simulink model "car_sim_for_student_r2015"  (R2022b)
settings: Solver=FixedStepAuto  StartTime=0.0  StopTime=40  FixedStep=0.001  RelTol=1e-3
InitFcn:
  | load('traj\traj_diySYSU.mat');
  | load('traj\sysu_standard.mat');
  | run lqr_nums.m
StopFcn:
  | run stopFunc.m
values from neighbouring files (symbols this model uses):
  k = lqr(A,B,Q,R)    [lqr_nums.m]
  map = ~map    [stopFunc.m]
undefined symbols (not defined in the file or in its folder): gray, out, trajSYSU
libraries: simulink x3, slpidlib x1
settings Model: Creator=Manny  LastModifiedBy=秦华谦
settings SolverCC: AlgebraicLoopSolver=LineSearch
settings OptimizationCC: LifeSpan=inf
settings DebuggingCC: UnconnectedInputMsg=warning  UnconnectedOutputMsg=warning  UnconnectedLineMsg=warning  SFExecutionAtInitializationDiag=none  SFMachineParentedDataDiag=warning  ArithmeticOperatorsInVariantConditions=warning
settings ModelReferenceCC: EnableRefExpFcnMdlSchedulingChecks=on
settings SFSimCC: CustomCodeUndefinedFunction=UseInterfaceOnly
settings CodeAppCC: StateflowObjectComments=on

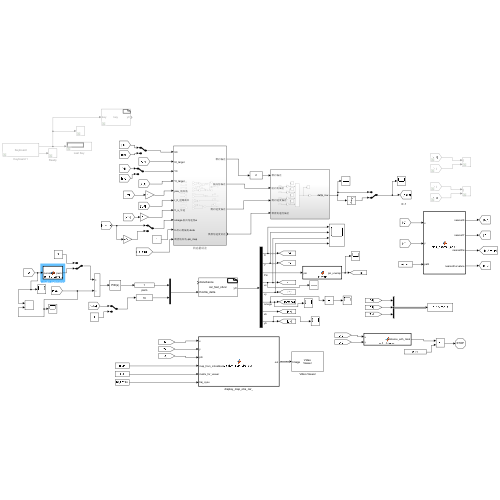
[thumbnail: Simulink's stored preview of the top-level diagram]
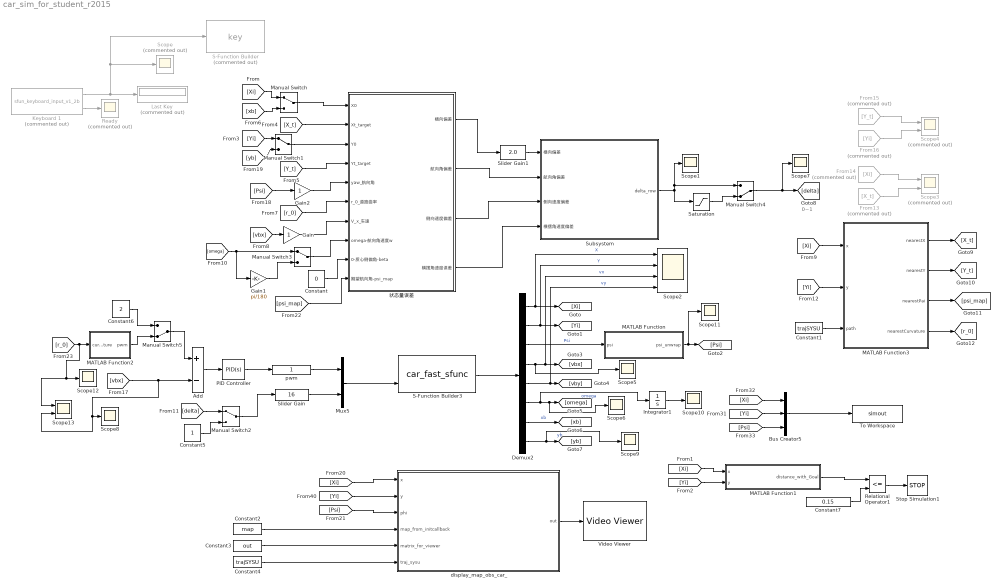
== system car_sim_for_student_r2015 ==
  note: 0~1
  Add : Sum  Inputs=+-
  Bus Creator5 : BusCreator  Inputs=3
  Constant : Constant  Value=0
  Constant1 : Constant  Value=trajSYSU
  Constant2 : Constant  Value=map
  Constant3 : Constant  Value=out
  Constant4 : Constant  Value=trajSYSU
  Constant5 : Constant
  Constant6 : Constant  Value=2
  Constant7 : Constant  Value=0.15
  Demux2 : Demux  Outputs=8
  From13 : From  Commented=on  GotoTag=X_t
  From14 : From  Commented=on  GotoTag=Xi
  From15 : From  Commented=on  GotoTag=Y_t
  From16 : From  Commented=on  GotoTag=Yi
  Gain : Gain
  Gain1 : Gain  Gain=pi/180
  Gain2 : Gain
  Integrator1 : Integrator
  Keyboard 1 : M-S-Function  Commented=on  FunctionName=sfun_keyboard_input_v1_2b  mask(Keyboard Input){}
      mask help: Keyboard Input
      mask Display: fprintf('Keyboard');
  Last Key : Display  Commented=on
  MATLAB Function : MATLAB Function  TreatAsAtomicUnit=on
  MATLAB Function1 : MATLAB Function  TreatAsAtomicUnit=on
  MATLAB Function2 : MATLAB Function  TreatAsAtomicUnit=on
  MATLAB Function3 : MATLAB Function  TreatAsAtomicUnit=on
  Manual Switch{,1..3} (4 alike) : ManualSwitch
  Manual Switch4 : ManualSwitch  CurrentSetting=0
  Manual Switch5 : ManualSwitch  CurrentSetting=0
  Mux5 : Mux  Inputs=2
  PID Controller : slpidlib/PID Controller  Controller=PID  Form=Parallel  TimeDomain=Continuous-time  UseExternalTs=off  SampleTime=-1  IntegratorMethod=Forward Euler  FilterMethod=Forward Euler  ControllerParametersSource=internal  P=2  I=0.3  UseKiTs=off  D=0.8  N=100  UseFilter=on  TunerSelectOption=Transfer Function Based (PID Tuner App)  InitialConditionSource=internal  InitialConditionForIntegrator=0  InitialConditionForFilter=0  DifferentiatorICPrevScaledInput=0  ExternalReset=none  TrackingMode=off  Kt=1  LimitOutput=off  SatLimitsSource=internal  UpperSaturationLimit=inf  LowerSaturationLimit=-inf  LinearizeAsGain=on  AntiWindupMode=none  Kb=1  LimitIntegrator=off  UpperIntegratorSaturationLimit=inf  LowerIntegratorSaturationLimit=-inf  POutMin=[]  POutMax=[]  IOutMin=[]  IOutMax=[]  DOutMin=[]  DOutMax=[]  NOutMin=[]  NOutMax=[]  SumOutMin=[]  SumOutMax=[]  SaturationOutMin=[]  SaturationOutMax=[]  PParamMin=[]  PParamMax=[]  IParamMin=[]  IParamMax=[]  DParamMin=[]  DParamMax=[]  NParamMin=[]  NParamMax=[]  KbParamMin=[]  KbParamMax=[]  KtParamMin=[]  KtParamMax=[]  KbOutMin=[]  KbOutMax=[]  KtOutMin=[]  KtOutMax=[]  IntegratorOutMin=[]  IntegratorOutMax=[]  FilterOutMin=[]  FilterOutMax=[]  SumI1OutMin=[]  SumI1OutMax=[]  SumI2OutMin=[]  SumI2OutMax=[]  SumI3OutMin=[]  SumI3OutMax=[]  SumI4OutMin=[]  SumI4OutMax=[]  SumDOutMin=[]  SumDOutMax=[]  DifferentiatorOutMin=[]  DifferentiatorOutMax=[]  FilterDiffOutCoefMin=[]  FilterDiffOutCoefMax=[]  ReciprocalOutMin=[]  ReciprocalOutMax=[]  SumDenOutMin=[]  SumDenOutMax=[]  SumNumOutMin=[]  SumNumOutMax=[]  DivideOutMin=[]  DivideOutMax=[]  UdiffTsProdOutMin=[]  UdiffTsProdOutMax=[]  NTsProdOutMin=[]  NTsProdOutMax=[]  UintegralTsProdOutMin=[]  UintegralTsProdOutMax=[]  UngainTsProdOutMin=[]  UngainTsProdOutMax=[]  ClampingZeroOutDataTypeStr=Inherit: Inherit via back propagation  ClampingZeroOutMin=[]  ClampingZeroOutMax=[]  FilterDenConstantOutDataTypeStr=Inherit: Inherit via back propagation  FilterDenConstantOutMin=[]  FilterDenConstantOutMax=[]  PCopyOutDataTypeStr=Inherit: Inherit via back propagation  PCopyOutMin=[]  PCopyOutMax=[]  NCopyOutDataTypeStr=Inherit: Inherit via back propagation  NCopyOutMin=[]  NCopyOutMax=[]  IntegratorContinuousStateAttributes=''  IntegratorStateMustResolveToSignalObject=off  IntegratorRTWStateStorageClass=Auto  FilterContinuousStateAttributes=''  FilterStateMustResolveToSignalObject=off  FilterRTWStateStorageClass=Auto  ParallelPVariant=InternalParameters  IdealPVariant=Disabled  IVariant=InternalParameters  DVariant=InternalParameters  IntegratorVariant=Continuous  SatVariant=Disabled  AWVariant=Passthrough  PCopyVariant=Disabled  TRVariant=Disabled  FdbkBlocksVariant=Forward  IdealPFdbkVariant=Disabled  SatFdbkVariant=Disabled  DerivativeFilterVariant=ContFilter  NVariant=InternalParameters  NCopyVariant=Disabled  FilterICVariant=InternalICsFilter  IntegratorICVariant=InternalICs  ExternalResetVariant=Disabled  TRSumVariant=Passthrough  SumFdbkVariant=Disabled  SumVariant=Sum_PID  TsampFilterVariant=InternalTs  TsampNgainVariant=Passthrough  TsampIntegralVariant=Passthrough  ExternalSaturationOutDataTypeStr=Inherit: Same as second input
  Ready : Scope  Commented=on
  Relational Operator1 : RelationalOperator  Operator=<=  OutDataTypeStr=boolean  InputSameDT=off
  S-Function Builder : S-Function  Commented=on  FunctionName=key  SFunctionModules=key_wrapper  SFunctionDeploymentMode=off  EnableBusSupport=off  mask(S-Function Builder){}
      mask help: Simulink:masks:SFunctionBuilder_MD
      mask init:
      | val = [[.9  0.75 0.75 1 1 .9 .9 1]',[1 1 0.75 0.75 .9 .9 1 .9]'];try , sys = get_param(gcb,'SfunBuilderFcnName');if isempty(sys), sys = get_param(gcb,'FunctionName'); end,catch, sys = get_param(gcb,'FunctionName'); end
      settings: CopyFcn=set_param(gcbh,'LinkStatus','none')  OpenFcn=sfunctionwizard(gcbh)
      mask Display:
      | plot(val(:,1),val(:,2))
      | disp(sys)
      | port_label('input',1,'key')
      | port_label('output',1,'y0')
  S-Function Builder3 : S-Function  FunctionName=car_fast_sfunc  SFunctionModules=car_fast_sfunc_wrapper  SFunctionDeploymentMode=off  EnableBusSupport=off  mask(S-Function Builder){}
      mask help: Simulink:masks:SFunctionBuilder_MD
      mask init: same as car_sim_for_student_r2015/S-Function Builder
      settings: CopyFcn=set_param(gcbh,'LinkStatus','none')  OpenFcn=sfunctionwizard(gcbh)
      mask Display:
      | plot(val(:,1),val(:,2))
      | disp(sys)
      | port_label('input',1,'disturbance')
      | port_label('input',2,'throttle_delta')
      | port_label('output',1,'y0')
  Saturation : Saturate  UpperLimit=1  LowerLimit=-1
  Scope : Scope  Commented=on
  Scope{1,5..12} (9 alike) : Scope
  Scope13 : Scope  NumInputPorts=2
  Scope2 : Scope  NumInputPorts=4
  Scope3 : Scope  Commented=on  NumInputPorts=2
  Scope4 : Scope  Commented=on  NumInputPorts=2
  Slider Gain : simulink/Math Operations/Slider Gain  gain=16  low=-20  high=20
  Slider Gain1 : simulink/Math Operations/Slider Gain  gain=2.0  low=0  high=2
  Stop Simulation1 : Stop
  Subsystem : Subsystem
  To Workspace : ToWorkspace  VariableName=simout  SaveFormat=Timeseries  SampleTime=-1
  Video Viewer : VideoViewer  colormapValue=gray(256)  FigPos=[295.4 757.2 1088 564]
  display_map_obs_car_ : MATLAB Function  TreatAsAtomicUnit=on
  pwm : simulink/Math Operations/Slider Gain  gain=1  low=-20  high=20
  状态量误差 : Subsystem
  wires:
  S-Function Builder3/1 -> Demux2/1
  Demux2/2 -> Scope2/2, [Yi]  "Y"
  Demux2/3 -> MATLAB Function/1(psi)  "Psi"
  Demux2/4 -> Scope5/1, Scope2/3, [vbx]  "vx"
  Demux2/5 -> Scope2/4, [vby]  "vy"
  Demux2/6 -> Integrator1/1, Scope6/1, [omega]  "omega"
  Demux2/7 -> [xb]  "xb"
  Demux2/8 -> Scope9/1, [yb]  "yb"
  MATLAB Function/1(psi_unwrap) -> Scope11/1, [Psi]
  [Yi] -> display_map_obs_car_/2(y)
  [Xi] -> display_map_obs_car_/1(x)
  [Psi] -> display_map_obs_car_/3(phi)
  display_map_obs_car_/1(out) -> Video Viewer/1
  Constant2/1 -> display_map_obs_car_/4(map_from_initcallback)
  Demux2/1 -> Scope2/1, [Xi]  "X"
  Constant3/1 -> display_map_obs_car_/5(matrix_for_viewer)
  pwm/1 -> Mux5/1
  Keyboard 1/1 -> S-Function Builder/1, Scope/1, Last Key/1
  Keyboard 1/2 -> Ready/1
  [Yi] -> Bus Creator5/2
  Bus Creator5/1 -> To Workspace/1
  [Psi] -> Bus Creator5/3
  [Xi] -> Bus Creator5/1
  Constant4/1 -> display_map_obs_car_/6(traj_sysu)
  Mux5/1 -> S-Function Builder3/2
  [Xi] -> MATLAB Function1/1(x)
  MATLAB Function1/1(distance_with_Goal) -> Relational Operator1/1
  Relational Operator1/1 -> Stop Simulation1/1
  Constant7/1 -> Relational Operator1/2
  [Yi] -> MATLAB Function1/2(y)
  状态量误差/1(横向偏差) -> Slider Gain1/1
  状态量误差/2(航向角偏差) -> Subsystem/2(航向角偏差)
  状态量误差/4(横摆角速度误差) -> Subsystem/4(横摆角速度偏差)
  状态量误差/3(侧向速度偏差) -> Subsystem/3(侧向速度偏差)
  Subsystem/1(delta_row) -> Saturation/1, Manual Switch4/1, Scope1/1
  [Xi] -> Manual Switch/1
  [Yi] -> Manual Switch1/1
  [X_t] -> 状态量误差/2(Xt_target)
  [Y_t] -> 状态量误差/4(Yt_target)
  [r_0] -> 状态量误差/6(r_0_道路曲率)
  Constant/1 -> 状态量误差/9(0-质心侧偏角-beta)
  [delta] -> Manual Switch2/1
  [vbx] -> Gain/1
  Constant1/1 -> MATLAB Function3/3(path)
  [Xi] -> MATLAB Function3/1(x)
  [Yi] -> MATLAB Function3/2(y)
  MATLAB Function3/1(nearestX) -> [X_t]
  MATLAB Function3/2(nearestY) -> [Y_t]
  MATLAB Function3/3(nearestPai) -> [psi_map]
  MATLAB Function3/4(nearestCurvature) -> [r_0]
  From13/1 -> Scope3/2
  From14/1 -> Scope3/1
  From15/1 -> Scope4/1
  From16/1 -> Scope4/2
  Slider Gain/1 -> Mux5/2
  Constant6/1 -> Manual Switch5/1
  Add/1 -> PID Controller/1
  PID Controller/1 -> pwm/1
  Gain/1 -> 状态量误差/7(V_x_车速)
  [vbx] -> Scope13/2, Scope8/1, Add/2
  [omega] -> Manual Switch3/1, Gain1/1
  Gain1/1 -> Manual Switch3/2
  Manual Switch4/1 -> Scope7/1, [delta]
  [xb] -> Manual Switch/2
  Manual Switch/1 -> 状态量误差/1(X0)
  [yb] -> Manual Switch1/2
  Manual Switch1/1 -> 状态量误差/3(Y0)
  [Psi] -> Gain2/1
  Integrator1/1 -> Scope10/1
  Manual Switch3/1 -> 状态量误差/8(omega-航向角速度w)
  [psi_map] -> 状态量误差/10(期望航向角-psi_map)
  Gain2/1 -> 状态量误差/5(yaw_航向角)
  Constant5/1 -> Manual Switch2/2
  Manual Switch2/1 -> Slider Gain/1
  Saturation/1 -> Manual Switch4/2
  [r_0] -> Scope12/1, Scope13/1, MATLAB Function2/1(curvature)
  Manual Switch5/1 -> Add/1
  MATLAB Function2/1(pwm) -> Manual Switch5/2
  Slider Gain1/1 -> Subsystem/1(横向偏差)

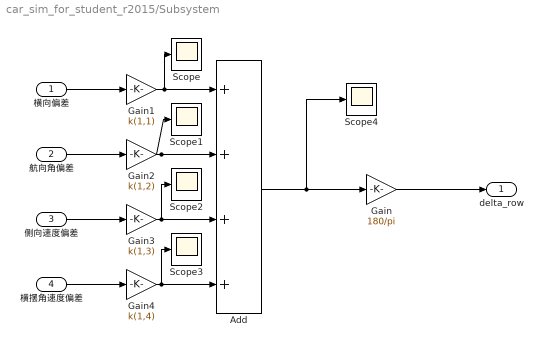
== system car_sim_for_student_r2015/Subsystem ==
  横向偏差 : Inport
  航向角偏差 : Inport  Port=2
  侧向速度偏差 : Inport  Port=3
  横摆角速度偏差 : Inport  Port=4
  Add : Sum  Inputs=++++
  Gain : Gain  Gain=180/pi
  Gain1 : Gain  Gain=k(1,1)
  Gain2 : Gain  Gain=k(1,2)
  Gain3 : Gain  Gain=k(1,3)
  Gain4 : Gain  Gain=k(1,4)
  Scope{,1..4} (5 alike) : Scope
  delta_row : Outport
  wires:
  横向偏差/1 -> Gain1/1
  航向角偏差/1 -> Gain2/1
  侧向速度偏差/1 -> Gain3/1
  横摆角速度偏差/1 -> Gain4/1
  Add/1 -> Scope4/1, Gain/1
  Gain/1 -> delta_row/1
  Gain1/1 -> Add/1, Scope/1
  Gain2/1 -> Scope1/1, Add/2
  Gain3/1 -> Add/3, Scope2/1
  Gain4/1 -> Scope3/1, Add/4

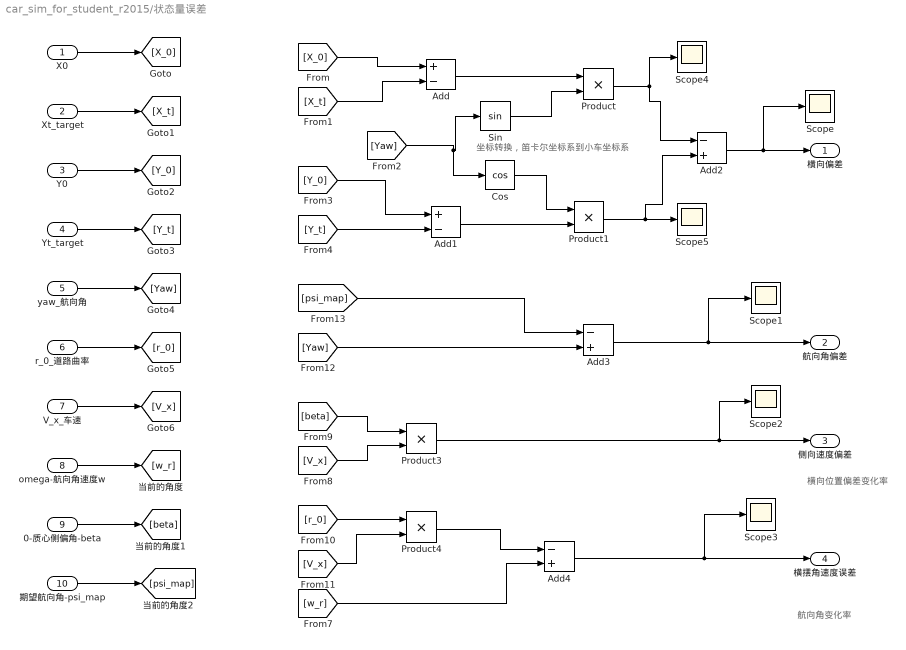
== system car_sim_for_student_r2015/状态量误差 ==
  note: 航向角变化率
  note: 横向位置偏差变化率
  note: 坐标转换，笛卡尔坐标系到小车坐标系
  X0 : Inport
  Xt_target : Inport  Port=2
  Y0 : Inport  Port=3
  Yt_target : Inport  Port=4
  yaw_航向角 : Inport  Port=5
  r_0_道路曲率 : Inport  Port=6
  V_x_车速 : Inport  Port=7
  omega-航向角速度w : Inport  Port=8
  0-质心侧偏角-beta : Inport  Port=9
  期望航向角-psi_map : Inport  Port=10
  Add : Sum  Inputs=+-
  Add1 : Sum  Inputs=+-
  Add2 : Sum  Inputs=-+
  Add3 : Sum  Inputs=-+
  Add4 : Sum  Inputs=-+
  Cos : Trigonometry  Operator=cos
  Product{,1,3..4} (4 alike) : Product
  Scope{,1..5} (6 alike) : Scope
  Sin : Trigonometry
  横向偏差 : Outport
  航向角偏差 : Outport  Port=2
  侧向速度偏差 : Outport  Port=3
  横摆角速度误差 : Outport  Port=4
  wires:
  X0/1 -> [X_0]
  Xt_target/1 -> [X_t]
  Y0/1 -> [Y_0]
  Yt_target/1 -> [Y_t]
  [X_0] -> Add/1
  [X_t] -> Add/2
  Add/1 -> Product/1
  yaw_航向角/1 -> [Yaw]
  [Yaw] -> Cos/1, Sin/1
  Sin/1 -> Product/2
  Cos/1 -> Product1/1
  [Y_0] -> Add1/1
  [Y_t] -> Add1/2
  Add1/1 -> Product1/2
  Product/1 -> Add2/1, Scope4/1
  Product1/1 -> Add2/2, Scope5/1
  Add2/1 -> Scope/1, 横向偏差/1
  r_0_道路曲率/1 -> [r_0]
  V_x_车速/1 -> [V_x]
  omega-航向角速度w/1 -> [w_r]
  [w_r] -> Add4/2
  Add3/1 -> Scope1/1, 航向角偏差/1
  [V_x] -> Product3/2
  0-质心侧偏角-beta/1 -> [beta]
  [beta] -> Product3/1
  Product3/1 -> Scope2/1, 侧向速度偏差/1
  [r_0] -> Product4/1
  [V_x] -> Product4/2
  Product4/1 -> Add4/1
  Add4/1 -> Scope3/1, 横摆角速度误差/1
  期望航向角-psi_map/1 -> [psi_map]
  [Yaw] -> Add3/2
  [psi_map] -> Add3/1

== matlab function car_sim_for_student_r2015/MATLAB Function1 ==
  data: x input; distance_with_Goal output; y input
function distance_with_Goal = cal_distance(x,y)
distance_with_Goal=sqrt((x-11.3)*(x-11.3)+(y-4.5)*(y-4.5))

== matlab function car_sim_for_student_r2015/display_map_obs_car_ ==
  settings: updateMethod=DISCRETE
  data: x input; y input; phi input; out output size=600,1200,3; map_from_initcallback input size=600,1200; matrix_for_viewer input; traj_sysu input
function out = display_map_obs_car_(x,y,phi,map_from_initcallback,matrix_for_viewer,traj_sysu)
    persistent data;
    persistent times;
    if isempty(data)
        times=1;
    else
        times=times+1;
    end

    % 地图长12m 宽6m   车长0.12 车宽0.06
    resolution = 0.01;
    map_long=12;
    map_wide=6;

    car_long=0.12;
    car_wide=0.06;

%     % 可视化地图
%     figure;
%     imagesc(map);%imagesc 可以将矩阵或数组的值映射到颜色图像中
%     colormap(flipud(gray));%colormap 将数据值映射到颜色空间中 colormap(flipud(gray)) 来设置颜色映射表为灰度图像。
    map=map_from_initcallback;    
    out=matrix_for_viewer;
    number_path=size(traj_sysu,2);
    for tmp=1:number_path
        traj_sysu_index=real2map([traj_sysu(1,tmp),traj_sysu(2,tmp)],map_wide,resolution);
        out(round(traj_sysu_index(1)+1/2),round(traj_sysu_index(2)+1/2),:)=[0,0,0];
    end
    x_now=x;%m  real视野坐标系,横着往右
    y_now=y;%m  real视野坐标系,竖着往上
    map_coord=real2map([x_now,y_now],map_wide,resolution);
    if isempty(data)
        data = zeros(99999, 2);
    else
        data(round(times/10)+1,:) = [map_coord(1),map_coord(2)];
        for times_disp_tmp=1:round(times/10)
            tmp_Data=data(times_disp_tmp,:);
            tmp_Data_next=data(times_disp_tmp+1,:);
%             out(round(tmp_Data(1,1)+1/2),round(tmp_Data(1,2)+1/2),:)=[0,0,1];

    
            vector=tmp_Data_next-tmp_Data;
            for t=0:0.025:1
                    new_point=tmp_Data+t*vector;
                    out(round(new_point(1)+1/2),round(new_point(2)+1/2),:)=[0,0,1];
                    out(round(new_point(1)+1/2),round(new_point(2)+1/2)-1,:)=[0,0,1];
                    out(round(new_point(1)+1/2),round(new_point(2)+1/2)+1,:)=[0,0,1];
            end

        end
    end



   
%     occ_or_not=get_occ_or_not(map_coord,map,resolution)
    occ_or_not=get_occ_or_not_Real([x_now,y_now],map_wide,map,resolution);
    l = car_long / resolution;
    w = car_wide / resolution;
    phi = phi; 




out=display_car(map_coord,phi,l,w,map,out);

%     axis equal;
%     axis off;
end

function occ_or_not=get_occ_or_not_Real(x_y,map_wide,map,resolution)
%round四舍五入 
map_coord=real2map(x_y,map_wide,resolution);
if(round(map_coord(1)+1/2)<1) ||(round(map_coord(1)+1/2)>600) ||(round(map_coord(2)+1/2)<1) ||(round(map_coord(2)+1/2)>1200)
    x_y
    disp('out of map');
end
 occ_or_not=map(round(map_coord(1)+1/2),round(map_coord(2)+1/2));
end
function occ_or_not=get_occ_or_not_map(map_coord,map,resolution)
%round四舍五入 
if(round(map_coord(1)+1/2)<1) ||(round(map_coord(1)+1/2)>600) ||(round(map_coord(2)+1/2)<1) ||(round(map_coord(2)+1/2)>1200)
    disp('out of map');
end
 occ_or_not=map(round(map_coord(1)+1/2),round(map_coord(2)+1/2));
end
function map_coord=real2map(x_y,map_wide,resolution)
    %地图向下是正x 向右是正y，
    % 因此在map上显示赛道小车障碍物的时候map_y直接取real世界的x, map_x需要把real_y反向并弄个静差
    map_coord=zeros(1,2);
    map_coord(1)=map_wide/ resolution-x_y(2)/ resolution;
    map_coord(2)=x_y(1)/ resolution ;
end

function matrix_for_viewer_new=display_car(map_coord,phi,l,w,map,matrix_for_viewer)
    %display是向右是x正，向下是y正
    pts = [
        map_coord(1)- [sin(phi)*l-cos(phi)*w, sin(phi)*l+cos(phi)*w,-sin(phi)*l+cos(phi)*w,-sin(phi)*l-cos(phi)*w]
        map_coord(2) + [cos(phi)*l+sin(phi)*w, cos(phi)*l-sin(phi)*w,-cos(phi)*l-sin(phi)*w,-cos(phi)*l+sin(phi)*w]
        
    ];
    map_index1=[round(pts(1,1)+1/2),round(pts(2,1)+1/2)];
    map_index2=[round(pts(1,2)+1/2),round(pts(2,2)+1/2)];
    map_index3=[round(pts(1,3)+1/2),round(pts(2,3)+1/2)];
    map_index4=[round(pts(1,4)+1/2),round(pts(2,4)+1/2)];

    matrix_for_viewer_new=matrix_for_viewer;
    %凸包，边缘线无碰撞则整体无碰撞
    have_somewhere_occ=0;
    vector_A_B=[map_index2(1)-map_index1(1),map_index2(2)-map_index1(2)];
    vector_A_D=[map_index4(1)-map_index1(1),map_index4(2)-map_index1(2)];
    for t1=0:0.025:1
        for t2=0:0.025:1
            new_point=map_index1+t1*vector_A_B+t2*vector_A_D;
            matrix_for_viewer_new(round(new_point(1)+0.5),round(new_point(2)+0.5),:)=[1,0,0];
            occ_or_not=map(round(new_point(1)+0.5),round(new_point(2)+0.5));
            if(occ_or_not==1)
               have_somewhere_occ=1;
           end
        end
    end
    if(have_somewhere_occ==1)
%         disp("collision!!");
    end
end

== matlab function car_sim_for_student_r2015/MATLAB Function ==
  data: psi input; psi_unwrap output
function psi_unwrap = unwrap(psi)

if ( psi > pi)
    psi = psi - 2*pi;
end

if( psi <= -pi)
    psi = psi + 2*pi;
end

psi_unwrap = psi;

== matlab function car_sim_for_student_r2015/MATLAB Function2 ==
  data: curvature input; pwm output
function pwm = adjust_by_curvature(curvature)
    % 设定一些常数
    max_output = 2.9;
    min_output = 0.3;
    max_curvature = 0.6;  
    
    % 计算反比例函数的值
    inv_proportional = 1 / abs(curvature);
    
    % 将反比例函数的值映射到0~1的范围内
    inv_proportional = inv_proportional / (1 / max_curvature);
    inv_proportional = min(max(inv_proportional, 0), 1);
    
    % 将0~1的值映射到0.3~3.3的范围内
    pwm = min_output + (max_output - min_output) * (inv_proportional);
end

== matlab function car_sim_for_student_r2015/MATLAB Function3 ==
  data: x input; nearestX output; y input; path input; nearestY output; nearestPai output; nearestCurvature output
function [nearestX, nearestY, nearestPai, nearestCurvature] = find_nearest_point(x, y, path)
% Initialize minDistance to a large value
minDistance = Inf;
nearestIndex = -1;

% Traverse through all points in the path
for i = 1:size(path, 2)
    % Calculate the Euclidean distance from the current point
    currentDistance = sqrt((path(1, i) - x)^2 + (path(2, i) - y)^2);
    % If this distance is less than the current minDistance, update minDistance
    % and nearestIndex
    if currentDistance < minDistance
        minDistance = currentDistance;
        nearestIndex = i;
    end
end

% If no point found, throw an error
if nearestIndex == -1
    error('No point found.');
end

% Return the parameters of the nearest point
nearestX = path(1, nearestIndex);
nearestY = path(2, nearestIndex);
nearestPai = path(3, nearestIndex);
nearestCurvature = path(4, nearestIndex);
end
